simulink model "AMR_main_24a"  (R2024a)
settings: configuration reference "SharedConfig" (kept outside this file)
values from neighbouring files (symbols this model uses):
  tstep = 0.001    [configuration_dictionary.sldd]
undefined symbols (not defined in the file or in its folder): Down, Pull, RTK_health_condition
libraries: speedgoatlib_IO60X_IO69X x11, tramontina_database_nvidialib x11, tramontina_database_curtislib x9, slrealtimeiplib x5, tramontina_database_curtis_mesalib x2, tramontina_database_moboticlib x2, speedgoatlib_IO691 x2, slrealtimeloglib x2, tramontina_database_sick_modbuslib x1, canmsglib x1, slrealtimeptplib x1
(part 1 of 2)
settings Model: DataDictionary=configuration_dictionary.sldd  SimulationMode=external  ExtModeEnableFloating=off  ExtModeTrigDuration=100000  Creator=matlab.cut  LastModifiedBy=matlab.cut
settings ConfigSetRef: SourceName=SharedConfig

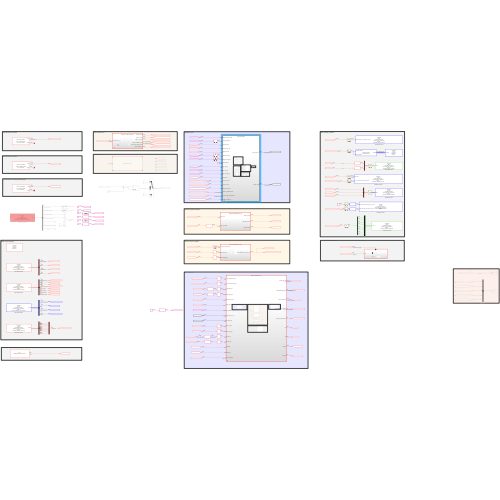
[thumbnail: Simulink's stored preview of the top-level diagram]
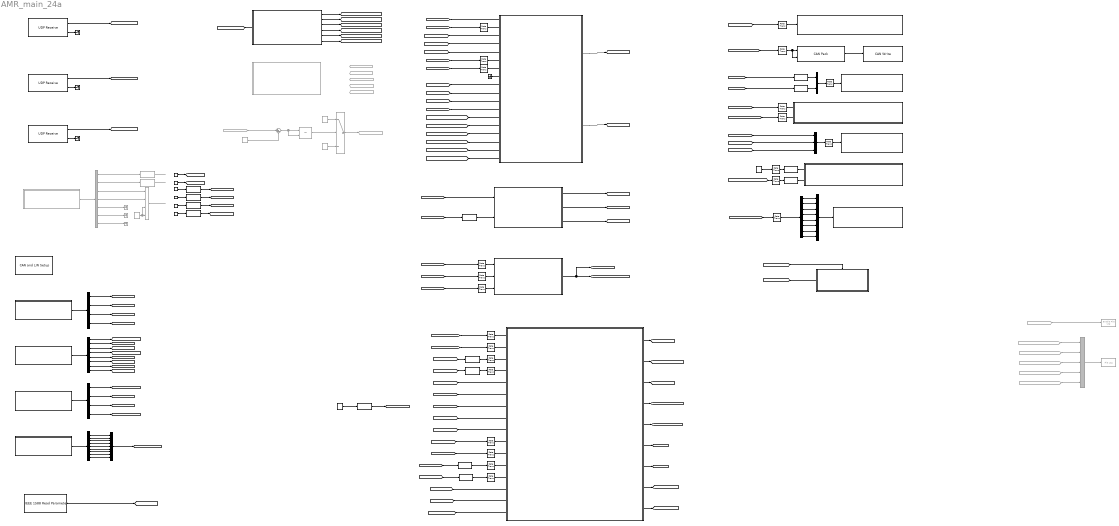
== system AMR_main_24a ==
  note: LidarLoc UPD Decoder
  note: Read UDP Data from Joystick
  note: Write UDP Data to LidarLoc Odometry
  note: Read System Time
  note: Motor Controll Untit
  note: guidance_unit
  note: operation_mode_selector
  note: vehicle_speed_readout
  note: CAN_output_interface
  note: CAN_input_interface
  note: Read UDP Data from Joystick
  note: gnss UPD Decoder
  note: Read UDP Data from ArduSimple Heading gnss
  Bus Creator : BusCreator  Inputs=8
  Bus Creator1 : BusCreator  Commented=on  Inputs=5
  Bus Creator2 : BusCreator  Inputs=2
  Bus Creator3 : BusCreator  Inputs=3
  Bus Selector1 : BusSelector  OutputSignals=ID1832_controller_status_RCUfront.controller_mode_front,ID1832_controller_status_RCUfront.MessageStatus.Status,ID1833_controller_status_RCUrear.controller_mode_rear,ID1833_controller_status_RCUrear.MessageStatus.Status
  Bus Selector6 : BusSelector  OutputSignals=ID1830_controller_status_left.controller_mode_left,ID1830_controller_status_left.MessageStatus.Status,ID1831_controller_status_right.MessageStatus.Status,ID1831_controller_status_right.controller_mode_right,ID422_curtis_feedback_message_left.motor_rpm_left,ID423_curtis_feedback_message_right.motor_rpm_right,ID934_curtis_encoder_left.rotor_position_left,ID935_curtis_encoder_right.rotor_position_rigth
  Bus Selector7 : BusSelector  Commented=on  OutputSignals=ID341_read_from_flexisoft.AuxEmEmergencia,ID341_read_from_flexisoft.AuxScannerInterrompido,ID341_read_from_flexisoft.EmergenciaFrontalDireita,ID341_read_from_flexisoft.EmergenciaFrontalEsquerda,ID341_read_from_flexisoft.EmergenciaTraseiraDireita,ID341_read_from_flexisoft.EmergenciaTraseiraEsquerda,ID341_read_from_flexisoft.MessageStatus.Status
  Bus Selector8 : BusSelector  OutputSignals=ID1459_feedback_word.MessageStatus.Status,ID1459_feedback_word.byte0,ID1459_feedback_word.byte1,ID1459_feedback_word.byte2,ID1459_feedback_word.byte3,ID1459_feedback_word.byte4,ID1459_feedback_word.byte5,ID1459_feedback_word.byte6,ID1459_feedback_word.byte7
  Bus Selector9 : BusSelector  OutputSignals=ID288_mobotic_feedback_pos.position_feedback,ID288_mobotic_feedback_pos.MessageStatus.Status,ID343_AMR_OperationMode.OperationMode,ID343_AMR_OperationMode.MessageStatus.Status
  CAN DB Parser Read 1 : Subsystem
      settings: OpenFcn=sg_can.OpenFcnRead;
      mask Help: eval('sg.utils.help.show(''io_main/refentry_ref_can_ofa_parsing_read'');')
      mask Display: disp('Speedgoat\nIO691\nCAN DB Parser Read\nModule ID: IO691 - Module ID 1\nChannel:  1\ntramontina_database_curtis_mesa.dbc ');
  CAN DB Parser Read 3 : Subsystem
      settings: OpenFcn=sg_can.OpenFcnRead;
      mask Help: eval('sg.utils.help.show(''io_main/refentry_ref_can_ofa_parsing_read'');')
      mask Display: disp('Speedgoat\nIO691\nCAN DB Parser Read\nModule ID: IO691 - Module ID 1\nChannel:  1\ntramontina_database_curtis.dbc ');
  CAN DB Parser Read 4 : Subsystem  Commented=on
      settings: OpenFcn=sg_can.OpenFcnRead;
      mask Help: eval('sg.utils.help.show(''io_main/refentry_ref_can_ofa_parsing_read'');')
      mask Display: disp('Speedgoat\nIO691\nCAN DB Parser Read\nModule ID: IO691 - Module ID 1\nChannel:  1\ntramontina_database_sick_modbus.dbc ');
  CAN DB Parser Read 7 : Subsystem
      settings: OpenFcn=sg_can.OpenFcnRead;
      mask Help: eval('sg.utils.help.show(''io_main/refentry_ref_can_ofa_parsing_read'');')
      mask Display: disp('Speedgoat\nIO691\nCAN DB Parser Read\nModule ID: IO691 - Module ID 1\nChannel:  1\ntramontina_database_mobotic.dbc ');
  CAN DB Parser Read 9 : Subsystem
      settings: OpenFcn=sg_can.OpenFcnRead;
      mask Help: eval('sg.utils.help.show(''io_main/refentry_ref_can_ofa_parsing_read'');')
      mask Display: disp('Speedgoat\nIO691\nCAN DB Parser Read\nModule ID: IO691 - Module ID 1\nChannel:  1\ntramontina_database_nvidia.dbc ');
  "CAN DB Parser Write " : Subsystem
      settings: OpenFcn=sg_can.OpenFcnWrite;
      mask Help: eval('sg.utils.help.show(''io_main/refentry_ref_can_ofa_parsing_write'');')
      mask Display: disp('Speedgoat\nIO691\nCAN DB Parser Write\nModule ID: IO691 - Module ID 1\nChannel:  1\ntramontina_database_nvidia.dbc ');
  CAN DB Parser Write 1 : Subsystem
      settings: OpenFcn=sg_can.OpenFcnWrite;
      mask Help: eval('sg.utils.help.show(''io_main/refentry_ref_can_ofa_parsing_write'');')
      mask Display: disp('Speedgoat\nIO691\nCAN DB Parser Write\nModule ID: IO691 - Module ID 1\nChannel:  1\ntramontina_database_nvidia.dbc ');
  CAN DB Parser Write 2 : Subsystem
      settings: OpenFcn=sg_can.OpenFcnWrite;
      mask Help: eval('sg.utils.help.show(''io_main/refentry_ref_can_ofa_parsing_write'');')
      mask Display: disp('Speedgoat\nIO691\nCAN DB Parser Write\nModule ID: IO691 - Module ID 1\nChannel:  1\ntramontina_database_curtis.dbc ');
  CAN DB Parser Write 3 : Subsystem
      settings: OpenFcn=sg_can.OpenFcnWrite;
      mask Help: eval('sg.utils.help.show(''io_main/refentry_ref_can_ofa_parsing_write'');')
      mask Display: disp('Speedgoat\nIO691\nCAN DB Parser Write\nModule ID: IO691 - Module ID 1\nChannel:  1\ntramontina_database_curtis.dbc ');
  CAN DB Parser Write 5 : Subsystem
      settings: OpenFcn=sg_can.OpenFcnWrite;
      mask Help: eval('sg.utils.help.show(''io_main/refentry_ref_can_ofa_parsing_write'');')
      mask Display: disp('Speedgoat\nIO691\nCAN DB Parser Write\nModule ID: IO691 - Module ID 1\nChannel:  1\ntramontina_database_nvidia.dbc ');
  CAN DB Parser Write 6 : Subsystem
      settings: OpenFcn=sg_can.OpenFcnWrite;
      mask Help: eval('sg.utils.help.show(''io_main/refentry_ref_can_ofa_parsing_write'');')
      mask Display: disp('Speedgoat\nIO691\nCAN DB Parser Write\nModule ID: IO691 - Module ID 1\nChannel:  1\ntramontina_database_mobotic.dbc ');
  CAN Pack2 : canmsglib/CAN Pack  MsgList=(none)  MsgName=CAN Msg  MsgIDType=Standard (11-bit identifier)  MsgIdentifier=0x120  MsgLength=8  Remote=off  ApplyMinMax=off  BusOutput=on  SignalInfo={ 'position_feedback', '0', '32', 'LE', 'signed', 'Standard', '0', '1', '0', '-inf', 'inf'; 'pulse_feedback', '32', '32', 'LE', 'signed', 'Standard', '0', '1', '0', '-Inf', 'Inf' }
      settings: DataFormat=manually specified signals
  CAN Write 2 : speedgoatlib_IO691/CAN Write   moduleType=IO691  id=1  channel=1  canType=CAN (HS)  messageType=CAN (HS)  useBusIn=on  numOfMsg=1  enableInput=off  enableStatusPort=off  ts=20e-3  initValues=[691 1 0.02 0 1 1 0 1 0 1]
      settings: SourceProductName=IO691
  "CAN and LIN Setup " : speedgoatlib_IO691/CAN and LIN Setup   moduleInitValues="[691    1    1   -1   -1]"  id=1  moduleType=IO691  pciSlot=-1  canChn1=CAN (HS)  canChn2=Disabled  canChn3=Disabled  canChn4=Disabled  linChn1=Disabled  linChn2=Disabled  canInitStructArray=[]  canTermStructArray=[]  gpioChnx=Disabled  canChn1InitValues="[2   2   8   1  16   3  19   2   2   5   2   0]"  arbBdrChn1=500 kBaud  clockDividerChn1=Enable  arbManBdrChn1=[8,1,16,3]  fdBdrChn1=5.0 MBaud  fdManBdrChn1=[2,2,5,2]  termResistor1=off  canChn2InitValues="[1   0   2   8  31   8  19   2   2   5   2   0]"  arbBdrChn2=1.0 MBaud  clockDividerChn2=Enable  arbManBdrChn2=[2,8,31,8]  fdBdrChn2=5.0 MBaud  fdManBdrChn2=[2,2,5,2]  termResistor2=off  canChn3InitValues="[1   0   2   8  31   8  19   2   2   5   2   0]"  arbBdrChn3=1.0 MBaud  clockDividerChn3=Enable  arbManBdrChn3=[2,8,31,8]  fdBdrChn3=5.0 MBaud  fdManBdrChn3=[2,2,5,2]  termResistor3=off  canChn4InitValues="[1   0   2   8  31   8  19   2   2   5   2   0]"  arbBdrChn4=1.0 MBaud  clockDividerChn4=Enable  arbManBdrChn4=[2,8,31,8]  fdBdrChn4=5.0 MBaud  fdManBdrChn4=[2,2,5,2]  termResistor4=off  linChn1InitValues="[0  9600]"  linBtrChn1=9600  linChn2InitValues="[0  9600]"  linBtrChn2=9600  doInitTermStruct="[0  5  0  0  0]"  parDoChannels=[1 2]  parDoVoltage=5  parDoInitValues=0  parDoReset=1  parNumOfDoS=0  parDiChannels=[3 4]  parDiVoltage=5  parDiPull=Pull-Down
      settings: LibrarySourceBlock=speedgoatlib_IO602_IO691/CAN and LIN Setup
  Cast{,1,4..9} (8 alike) : DataTypeConversion  OutDataTypeStr=boolean  SaturateOnIntegerOverflow=off  RndMeth=Floor
  Cast To Boolean : DataTypeConversion  Commented=on  OutDataTypeStr=boolean  SaturateOnIntegerOverflow=off  RndMeth=Floor
  Cast To Boolean1 : DataTypeConversion  Commented=on  OutDataTypeStr=boolean  SaturateOnIntegerOverflow=off  RndMeth=Floor
  Cast10 : DataTypeConversion  OutDataTypeStr=double  SaturateOnIntegerOverflow=off  RndMeth=Floor
  Cast11 : DataTypeConversion  OutDataTypeStr=double  SaturateOnIntegerOverflow=off  RndMeth=Floor
  Cast13 : DataTypeConversion  OutDataTypeStr=int64  SaturateOnIntegerOverflow=off  RndMeth=Floor
  Cast14 : DataTypeConversion  OutDataTypeStr=int64  SaturateOnIntegerOverflow=off  RndMeth=Floor
  Cast2 : DataTypeConversion  OutDataTypeStr=single  SaturateOnIntegerOverflow=off  RndMeth=Floor
  Cast3 : DataTypeConversion  OutDataTypeStr=single  SaturateOnIntegerOverflow=off  RndMeth=Floor
  Constant : Constant  OutDataTypeStr=boolean
  Constant1 : Constant
  Constant10 : Constant  Commented=on
  Constant2 : Constant
  Constant3 : Constant  Value=0
  Constant4 : Constant
  Constant5 : Constant  Value=0
  Constant8 : Constant  Commented=on
  Constant9 : Constant  Commented=on  Value=0
  Demux1 : Demux  Outputs=8
  Enable File Log : slrealtimeloglib/Enable File Log  Commented=on
  Enabled Subsystem : Subsystem  TreatAsAtomicUnit=on
  File Log : slrealtimeloglib/File Log  Commented=on  decimation=1  inputProcessing=Elements as channels (sample based)
  From46 : From  Commented=on  GotoTag=GPS_RTKstatus
  From48 : From  Commented=on  GotoTag=LidarLoc_result_x
  From52 : From  Commented=on  GotoTag=LidarLoc_result_y
  From54 : From  Commented=on  GotoTag=LidarLoc_result_yaw
  From55 : From  Commented=on  GotoTag=LidarLoc_localization_status
  From56 : From  Commented=on  GotoTag=LidarLoc_map_matching_status
  From57 : From  Commented=on  GotoTag=AMR_auto_mode
  Goto22 : Goto  Commented=on  GotoTag=GPS_rtk_trustness
  Goto25 : Goto  Commented=on  GotoTag=GPS_RTKstatus
  Goto3 : Goto  Commented=on  GotoTag=gnss_lat_deg
  Goto4 : Goto  Commented=on  GotoTag=gnss_lon_deg
  Goto5 : Goto  Commented=on  GotoTag=gnss_heading_deg
  Goto9 : Goto  Commented=on  GotoTag=GPS_GNSSfix
  Ground : Ground
  IEEE 1588 Read Parameter : slrealtimeptplib/IEEE 1588 Read Parameter  Priority=1  ID=1  param=1. System time (nanosecond)  sample_time=tstep
  Integrator1 : Integrator  Commented=on  ExternalReset=either  UpperSaturationLimit=1  LowerSaturationLimit=0  WrappedStateUpperValue=30  WrappedStateLowerValue=0
  Model : ModelReference  ModelNameDialog=deployAMR_stateflow.slx  SimulationMode=Normal  ModelReferenceVersion=3.78
  Model1 : ModelReference  ModelNameDialog=AMR_OperationModeSelector_24a.slx  SimulationMode=Normal  ModelReferenceVersion=2.14
  Model2 : ModelReference  ModelNameDialog=AMR_LidarLoc_UDP_decoder_24a.slx  SimulationMode=Normal  ModelReferenceVersion=5.26
  Model3 : ModelReference  ModelNameDialog=AMR_VehicleSpeedReadout_24a.slx  SimulationMode=Normal  ModelReferenceVersion=2.16
  Model4 : ModelReference  ModelNameDialog=AMR_MotorControlUnit_24a.slx  SimulationMode=Normal  ModelReferenceVersion=2.51
      settings: PortSchema="{\"entries\":[{\"content\":{\"sides\":[{\"content\":{\"connectorIds\":[\"In1\",\"In2\",\"In3\",\"In4\",\"In6\",\"In7\",\"In8\",\"In9\",\"In10\",\"In11\",\"In12\",\"In13\",\"In14\",\"In15\",\"In5\",\"In16\"]},\"type\":\"ConnectorPlacement.EquallySpacedRectSide\",\"uuid\":\"7c2b178d-2b94-42de-b877-cc3b9587523f\"},{\"content\":{\"connectorIds\":[\"Out1\",\"Out2\",\"Out3\",\"Out4\",\"Out5\",\"Out6\",\"Out7\",\"Out8\",\"Out9\"],\"side\":\"RIGHT\"},\"type\":\"ConnectorPlacement.EquallySpacedRectSide\",\"uuid\":\"578e4da8-0cd4-4538-9680-61a080b2bcd8\"},{\"content\":{\"side\":\"TOP\"},\"type\":\"ConnectorPlacement.EquallySpacedRectSide\",\"uuid\":\"8fde1a66-cc00-48a8-a863-0a641ec024c7\"}]},\"type\":\"ConnectorPlacement.EquallySpacedConnector\",\"uuid\":\"3439c5b0-61a5-4e62-aad1-c2c681181905\"}],\"packageUris\":[\"http://schema.mathworks.com/mf0/Connector/R2020b\"],\"version\":\"1.0\"}"
  Model5 : ModelReference  Commented=on  SimulationMode=Normal
  Mux : Mux  Inputs=9
  OR : Logic  Commented=on  Operator=OR  Inputs=4  AllPortsSameDT=off  OutDataTypeStr=boolean
  Rate Transition{,1..2,6,9..10,15,22..24,26,28..29,32,38,40..44} (20 alike) : RateTransition
  Rate Transition11 : RateTransition  OutPortSampleTimeOpt=Inherit
  Rate Transition12 : RateTransition  Deterministic=off
  Rate Transition21 : RateTransition  OutPortSampleTimeOpt=Inherit
  Sum1 : Sum  Commented=on  Inputs=|+-
  Switch2 : Switch  Commented=on  Criteria=u2 > Threshold  Threshold=RTK_health_condition  SaturateOnIntegerOverflow=off  InputSameDT=off
  Terminator : Terminator  Commented=on
  Terminator1 : Terminator  Commented=on
  Terminator2 : Terminator  Commented=on
  Terminator3 : Terminator
  Terminator4 : Terminator
  Terminator5 : Terminator
  UDP Receive : slrealtimeiplib/UDP Receive  useHostTargetConn=off  ipAddress=10.200.83.53  localPort=25000  rcvWidth=36  rcvFmAny=off  fmAddress='10.200.83.57'  sampleTime=tstep  enableMessage=off  maxPackets=1
  UDP Receive1 : slrealtimeiplib/UDP Receive  useHostTargetConn=off  ipAddress=10.200.83.53  localPort=5010  rcvWidth=56  rcvFmAny=on  fmAddress='10.200.83.57'  sampleTime=tstep  enableMessage=off  maxPackets=1
  UDP Receive2 : slrealtimeiplib/UDP Receive  useHostTargetConn=off  ipAddress=10.200.83.53  localPort=5015  rcvWidth=36  rcvFmAny=off  fmAddress='10.200.83.57'  sampleTime=tstep  enableMessage=off  maxPackets=1
  Zero : Constant  Commented=on  Value=0  OutDataTypeStr=Inherit: Inherit via back propagation
  Zero1 : Constant  Value=0  OutDataTypeStr=Inherit: Inherit via back propagation
  Zero2 : Constant  Value=0  OutDataTypeStr=Inherit: Inherit via back propagation
  wires:
  Rate Transition32/1 -> CAN DB Parser Write 5/1(ID289_mobotic_error_flag.steering_unit_error)
  Rate Transition28/1 -> Cast2/1
  [AMR_speed_to_CAN_m_per_sec] -> Rate Transition29/1
  Zero2/1 -> Rate Transition28/1
  CAN Pack2/1 -> CAN Write 2/1
  Bus Creator2/1 -> Rate Transition15/1
  [rws] -> Cast11/1  "rws"
  Cast10/1 -> Bus Creator2/1
  Rate Transition6/1 -> CAN DB Parser Write 3/2(ID0_curtis_input_operational.pre_operational)
  Bus Creator3/1 -> Rate Transition12/1
  [steering_unit_error] -> Rate Transition32/1
  Rate Transition10/1 -> CAN Pack2/2, CAN Pack2/1
  Rate Transition29/1 -> Cast3/1
  [curtis_controller_into_operation] -> Rate Transition6/1
  [lws] -> Cast10/1  "lws"
  Cast11/1 -> Bus Creator2/2
  [steering_unit_theta_position] -> Rate Transition10/1
  [controller_enable_flag] -> Rate Transition24/1
  Rate Transition15/1 -> CAN DB Parser Write 2/1(CAN Tx)
  Rate Transition24/1 -> CAN DB Parser Write 3/1(Enable Input)
  [interlock] -> Rate Transition44/1
  [emergency] -> Rate Transition43/1
  [scanner_blocked] -> Rate Transition42/1
  Rate Transition44/1 -> Model/2
  [gate_closed_ahead] -> Model/1
  Model/1 -> [target_speed_m_per_s]  "target_speed_m_s"
  Model/2 -> [sw_target_angle]  "sw_target_angle"
  Cast4/1 -> Model1/2
  Model1/1 -> [AMR_idle_mode]
  Model1/2 -> [AMR_manual_mode]
  Model1/3 -> [AMR_auto_mode]
  [curtis_controller_mode_left] -> Rate Transition21/1
  Rate Transition22/1 -> Model4/3
  Rate Transition21/1 -> Model4/1
  Rate Transition23/1 -> Model4/4
  Rate Transition11/1 -> Model4/2
  [curtis_status_right] -> Cast1/1
  [curtis_status_left] -> Cast5/1
  [curtis_controller_mode_right] -> Rate Transition11/1
  [motor_rpm_right] -> Rate Transition41/1
  [steering_unit_pos] -> Rate Transition38/1
  [motor_rpm_left] -> Rate Transition40/1
  Model3/1 -> [AMR_speed_to_CAN_m_per_sec], [AMR_speed]
  Rate Transition38/1 -> Model3/1
  Rate Transition41/1 -> Model3/3
  Rate Transition40/1 -> Model3/2
  [motor_rpm_left] -> Rate Transition26/1
  [motor_rpm_right] -> Rate Transition9/1
  Cast2/1 -> CAN DB Parser Write 1/1(ID290_AMR_vehicle_speed.speed_m_per_min)
  Cast3/1 -> CAN DB Parser Write 1/2(ID290_AMR_vehicle_speed.speed_m_per_s)
  [AMR_idle_mode] -> Bus Creator3/1
  [AMR_auto_mode] -> Bus Creator3/3
  [AMR_manual_mode] -> Bus Creator3/2
  Cast5/1 -> Rate Transition22/1
  Cast1/1 -> Rate Transition23/1
  Rate Transition12/1 -> "CAN DB Parser Write "/1(CAN Tx)
  [oper_mode] -> Model1/1
  [oper_mode_status] -> Cast4/1
  Model4/1 -> [steering_unit_error]  "steering_unit_error"
  Model4/7 -> [rws]
  Bus Selector7/4 -> OR/2  "<EmergenciaFrontalEsquerda>"
  Zero/1 -> OR/3, OR/4
  Bus Selector9/4 -> [oper_mode_status]  "<Status>"
  Bus Selector9/3 -> [oper_mode]  "<OperationMode>"
  Cast To Boolean/1 -> ?
  CAN DB Parser Read 9/1(CAN Rx) -> Bus Selector9/1
  Bus Selector9/1 -> [steering_unit_pos]  "<position_feedback>"
  Bus Selector7/7 -> Terminator/1  "<Status>"
  Cast To Boolean1/1 -> ?
  Bus Selector7/1 -> Cast To Boolean/1  "<AuxEmEmergencia>"
  CAN DB Parser Read 4/1(CAN Rx) -> Bus Selector7/1
  CAN DB Parser Read 7/1(CAN Rx) -> Bus Selector8/1
  OR/1 -> ?  "emergency"
  Bus Selector7/2 -> Cast To Boolean1/1  "<AuxScannerInterrompido>"
  Bus Selector7/6 -> Terminator1/1  "<EmergenciaTraseiraEsquerda>"
  Bus Selector7/3 -> OR/1  "<EmergenciaFrontalDireita>"
  Bus Selector7/5 -> Terminator2/1  "<EmergenciaTraseiraDireita>"
  Bus Selector9/2 -> [steering_unit_status]  "<Status>"
  From46/1 -> Sum1/1
  Constant10/1 -> Sum1/2
  Constant9/1 -> Switch2/3
  Switch2/1 -> Goto22/1  "rtk_trustness"
  Integrator1/1 -> Switch2/2  "rtk_integrator"
  Constant8/1 -> Switch2/1
  Sum1/1 -> Integrator1/2, Integrator1/1  "rtk_diff"
  Rate Transition9/1 -> Model4/12
  [mobotic_Rx] -> Model4/5
  [AMR_manual_mode] -> Model4/6
  [AMR_auto_mode] -> Model4/7
  Demux1/8 -> Bus Creator/8
  Demux1/6 -> Bus Creator/6
  Demux1/4 -> Bus Creator/4
  Demux1/3 -> Bus Creator/3
  Demux1/5 -> Bus Creator/5
  Bus Creator/1 -> CAN DB Parser Write 6/1(CAN Tx)
  Demux1/7 -> Bus Creator/7
  [CANOpenMessage_Output] -> Rate Transition/1
  Rate Transition/1 -> Demux1/1
  Demux1/2 -> Bus Creator/2
  Demux1/1 -> Bus Creator/1
  Mux/1 -> [mobotic_Rx]  "mobotic_Rx"
  Bus Selector8/1 -> Mux/1  "<Status>"
  Bus Selector8/2 -> Mux/2  "<byte0>"
  Bus Selector8/3 -> Mux/3  "<byte1>"
  Bus Selector8/4 -> Mux/4  "<byte2>"
  Bus Selector8/5 -> Mux/5  "<byte3>"
  Bus Selector8/6 -> Mux/6  "<byte4>"
  Bus Selector8/7 -> Mux/7  "<byte5>"
  Bus Selector8/8 -> Mux/8  "<byte6>"
  Bus Selector8/9 -> Mux/9  "<byte7>"
  UDP Receive/2 -> Terminator4/1
  Model4/6 -> [lws]
  Model4/5 -> [steering_unit_theta_position]
  Model4/2 -> [CANOpenMessage_Output]  "CANOpenMessage_Output"
  Model4/3 -> [controller_enable_flag]  "controller_enable_flag"
  Model4/4 -> [curtis_controller_into_operation]  "curtis_controller_into_operation"
  Bus Selector1/3 -> [curtis_status_rear]  "<controller_mode_rear>"
  Bus Selector1/1 -> [curtis_controller_mode_front]  "<controller_mode_front>"
  Bus Selector1/4 -> [curtis_controller_mode_rear]  "<Status>"
  Bus Selector1/2 -> [curtis_status_front]  "<Status>"
  CAN DB Parser Read 1/1(CAN Rx) -> Bus Selector1/1
  Model4/8 -> [send_flag_odometry]
  Model4/9 -> [udp_string_odometry]
  [send_flag_odometry] -> Enabled Subsystem/Trigger  "sick_odometry_send_flag"
  [udp_string_odometry] -> Enabled Subsystem/1(data)  "udp_string"
  IEEE 1588 Read Parameter/1 -> [timestamp]  "output"
  [timestamp] -> Model4/15
  Bus Selector6/6 -> [motor_rpm_right]  "<motor_rpm_right>"
  Bus Selector6/5 -> [motor_rpm_left]  "<motor_rpm_left>"
  CAN DB Parser Read 3/1(CAN Rx) -> Bus Selector6/1
  Bus Selector6/8 -> [motor_encoder_right]  "<rotor_position_rigth>"
  Bus Selector6/2 -> [curtis_status_left]  "<Status>"
  Bus Selector6/4 -> [curtis_controller_mode_right]  "<controller_mode_right>"
  Bus Selector6/3 -> [curtis_status_right]  "<Status>"
  Bus Selector6/7 -> [motor_encoder_left]  "<rotor_position_left>"
  Bus Selector6/1 -> [curtis_controller_mode_left]  "<controller_mode_left>"
  Cast14/1 -> Rate Transition2/1
  Cast13/1 -> Rate Transition1/1  "encoder_left_int"
  [motor_encoder_right] -> Cast14/1
  [motor_encoder_left] -> Cast13/1  "encoder_left_double"
  Rate Transition1/1 -> Model4/13
  Rate Transition2/1 -> Model4/14
  UDP Receive/1 -> [udp_from_joystick]  "joy_axes"
  [udp_from_joystick] -> Model4/16
  [GPS_GNSSfix] -> Model4/8
  [target_speed_m_per_s] -> Model4/9
  [sw_target_angle] -> Model4/10
  Rate Transition26/1 -> Model4/11
  UDP Receive1/1 -> [udp_from_lidarLoc]  "udp_from_lidarLoc"
  UDP Receive1/2 -> Terminator3/1
  [udp_from_lidarLoc] -> Model2/1
  Model2/5 -> [LidarLoc_map_matching_status]
  Model2/4 -> [LidarLoc_localization_status]
  Model2/3 -> [LidarLoc_result_yaw]
  Model2/2 -> [LidarLoc_result_y]
  ? -> ?
  UDP Receive2/1 -> [udp_from_gnss]  "joy_axes"
  Constant/1 -> Cast/1
  Bus Creator1/1 -> File Log/1
  From48/1 -> Bus Creator1/1
  From52/1 -> Bus Creator1/2
  From54/1 -> Bus Creator1/3
  From55/1 -> Bus Creator1/4
  From56/1 -> Bus Creator1/5
  From57/1 -> Enable File Log/1  "auto_mode"
  Cast/1 -> [GPS_GNSSfix]
  Constant1/1 -> Cast6/1
  Constant3/1 -> Cast7/1
  Constant2/1 -> Cast8/1
  Model2/6 -> [LidarLoc_telegram_ok]
  Model2/1 -> [LidarLoc_result_x]
  [AMR_manual_mode] -> Model/4
  [AMR_auto_mode] -> Model/5
  [AMR_idle_mode] -> Model/3
  Rate Transition42/1 -> Model/6
  Rate Transition43/1 -> Model/7
  Ground/1 -> Model/8
  [gnss_lat_deg] -> Model/9
  [gnss_lon_deg] -> Model/10
  [gnss_heading_deg] -> Model/11
  [AMR_speed] -> Model/12
  [LidarLoc_result_x] -> Model/13
  [LidarLoc_result_y] -> Model/14
  [LidarLoc_result_yaw] -> Model/15
  [LidarLoc_localization_status] -> Model/16
  [LidarLoc_map_matching_status] -> Model/17
  [LidarLoc_telegram_ok] -> Model/18
  UDP Receive2/2 -> Terminator5/1
  Constant4/1 -> [one]
  Constant5/1 -> [nulo]
  Cast6/1 -> [interlock]
  Cast8/1 -> [emergency]
  Cast7/1 -> [scanner_blocked]
  Zero1/1 -> Cast9/1
  Cast9/1 -> [gate_closed_ahead]

== system AMR_main_24a/CAN DB Parser Read 1 ==
  ReadSubsystem : Subsystem
  UnpackSubsystem : Subsystem
  CAN Rx : Outport
  wires:
  ReadSubsystem/1(Raw_Rx) -> UnpackSubsystem/1(Unpack_In)
  ReadSubsystem/2(Status_Rx) -> UnpackSubsystem/2(Status Inport)
  UnpackSubsystem/1(Unpack_Out) -> CAN Rx/1

== system AMR_main_24a/CAN DB Parser Read 3 ==
  ReadSubsystem : Subsystem
  UnpackSubsystem : Subsystem
  CAN Rx : Outport
  wires:
  ReadSubsystem/1(Raw_Rx) -> UnpackSubsystem/1(Unpack_In)
  ReadSubsystem/2(Status_Rx) -> UnpackSubsystem/2(Status Inport)
  UnpackSubsystem/1(Unpack_Out) -> CAN Rx/1

== system AMR_main_24a/CAN DB Parser Read 4 ==
  ReadSubsystem : Subsystem
  UnpackSubsystem : Subsystem
  CAN Rx : Outport
  wires:
  ReadSubsystem/1(Raw_Rx) -> UnpackSubsystem/1(Unpack_In)
  ReadSubsystem/2(Status_Rx) -> UnpackSubsystem/2(Status Inport)
  UnpackSubsystem/1(Unpack_Out) -> CAN Rx/1

== system AMR_main_24a/CAN DB Parser Read 7 ==
  ReadSubsystem : Subsystem
  UnpackSubsystem : Subsystem
  CAN Rx : Outport
  wires:
  ReadSubsystem/1(Raw_Rx) -> UnpackSubsystem/1(Unpack_In)
  ReadSubsystem/2(Status_Rx) -> UnpackSubsystem/2(Status Inport)
  UnpackSubsystem/1(Unpack_Out) -> CAN Rx/1

== system AMR_main_24a/CAN DB Parser Read 9 ==
  ReadSubsystem : Subsystem
  UnpackSubsystem : Subsystem
  CAN Rx : Outport
  wires:
  ReadSubsystem/1(Raw_Rx) -> UnpackSubsystem/1(Unpack_In)
  ReadSubsystem/2(Status_Rx) -> UnpackSubsystem/2(Status Inport)
  UnpackSubsystem/1(Unpack_Out) -> CAN Rx/1

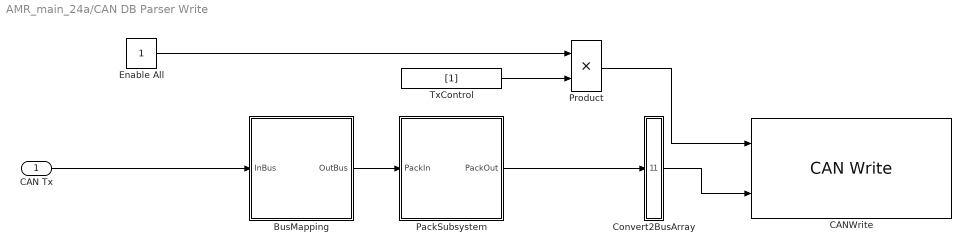
== system AMR_main_24a/CAN DB Parser Write  ==
  CAN Tx : Inport
  BusMapping : Subsystem
  CANWrite : speedgoatlib_IO60X_IO69X/CAN/CAN Write   moduleType=IO691  id=1  channel=1  canType=CAN (HS)  messageType=CAN (HS)  useBusIn=on  numOfMsg=1  enableInput=on  enableStatusPort=off  ts=500e-3  initValues=[691 1 0.5 0 1 1 0 1 1 1]
  Convert2BusArray : Subsystem
  Enable All : Constant  OutDataTypeStr=boolean
  PackSubsystem : Subsystem
  Product : Product  OutDataTypeStr=uint32
  TxControl : Constant  Value=[1]  OutDataTypeStr=uint32
  wires:
  PackSubsystem/1(PackOut) -> Convert2BusArray/1(InBus)
  Convert2BusArray/1(BusArrayOut) -> CANWrite/2
  Product/1 -> CANWrite/1
  TxControl/1 -> Product/2
  Enable All/1 -> Product/1
  CAN Tx/1 -> BusMapping/1(InBus)
  BusMapping/1(OutBus) -> PackSubsystem/1(PackIn)

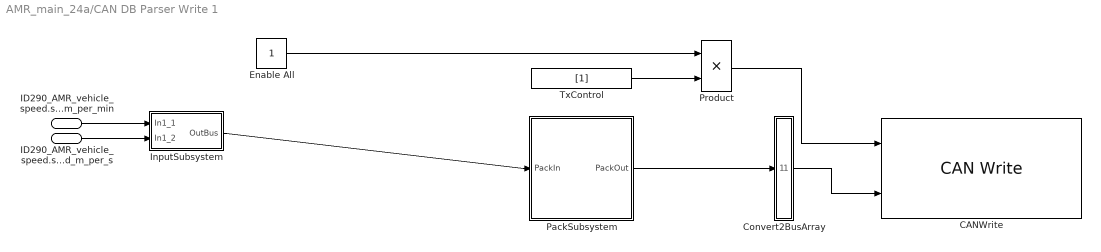
== system AMR_main_24a/CAN DB Parser Write 1 ==
  ID290_AMR_vehicle_speed.speed_m_per_min : Inport
  ID290_AMR_vehicle_speed.speed_m_per_s : Inport  Port=2
  CANWrite : speedgoatlib_IO60X_IO69X/CAN/CAN Write   moduleType=IO691  id=1  channel=1  canType=CAN (HS)  messageType=CAN (HS)  useBusIn=on  numOfMsg=1  enableInput=on  enableStatusPort=off  ts=50e-3  initValues=[691 1 0.05 0 1 1 0 1 1 1]
  Convert2BusArray : Subsystem
  Enable All : Constant  OutDataTypeStr=boolean
  InputSubsystem : Subsystem
  PackSubsystem : Subsystem
  Product : Product  OutDataTypeStr=uint32
  TxControl : Constant  Value=[1]  OutDataTypeStr=uint32
  wires:
  PackSubsystem/1(PackOut) -> Convert2BusArray/1(InBus)
  Convert2BusArray/1(BusArrayOut) -> CANWrite/2
  Product/1 -> CANWrite/1
  TxControl/1 -> Product/2
  Enable All/1 -> Product/1
  ID290_AMR_vehicle_speed.speed_m_per_min/1 -> InputSubsystem/1(In1_1)
  ID290_AMR_vehicle_speed.speed_m_per_s/1 -> InputSubsystem/2(In1_2)
  InputSubsystem/1(OutBus) -> PackSubsystem/1(PackIn)

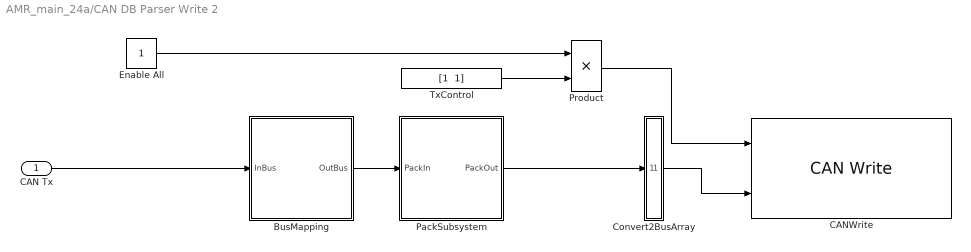
== system AMR_main_24a/CAN DB Parser Write 2 ==
  CAN Tx : Inport
  BusMapping : Subsystem
  CANWrite : speedgoatlib_IO60X_IO69X/CAN/CAN Write   moduleType=IO691  id=1  channel=1  canType=CAN (HS)  messageType=CAN (HS)  useBusIn=on  numOfMsg=2  enableInput=on  enableStatusPort=off  ts=10e-3  initValues=[691 1 0.01 0 1 1 0 2 1 1]
  Convert2BusArray : Subsystem
  Enable All : Constant  OutDataTypeStr=boolean
  PackSubsystem : Subsystem
  Product : Product  OutDataTypeStr=uint32
  TxControl : Constant  Value="[1  1]"  OutDataTypeStr=uint32
  wires:
  PackSubsystem/1(PackOut) -> Convert2BusArray/1(InBus)
  Convert2BusArray/1(BusArrayOut) -> CANWrite/2
  Product/1 -> CANWrite/1
  TxControl/1 -> Product/2
  Enable All/1 -> Product/1
  CAN Tx/1 -> BusMapping/1(InBus)
  BusMapping/1(OutBus) -> PackSubsystem/1(PackIn)

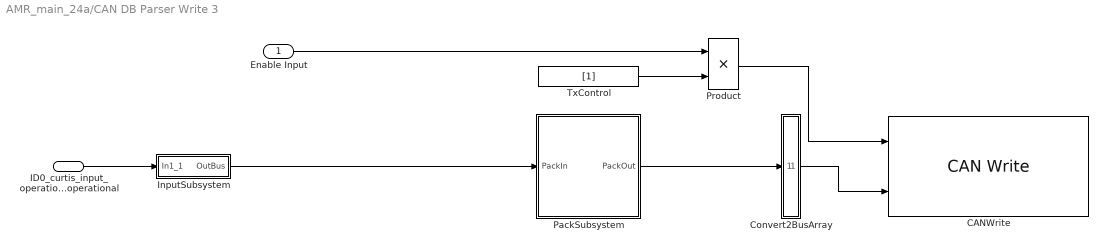
== system AMR_main_24a/CAN DB Parser Write 3 ==
  Enable Input : Inport  OutDataTypeStr=boolean
  ID0_curtis_input_operational.pre_operational : Inport  Port=2
  CANWrite : speedgoatlib_IO60X_IO69X/CAN/CAN Write   moduleType=IO691  id=1  channel=1  canType=CAN (HS)  messageType=CAN (HS)  useBusIn=on  numOfMsg=1  enableInput=on  enableStatusPort=off  ts=500e-3  initValues=[691 1 0.5 0 1 1 0 1 1 1]
  Convert2BusArray : Subsystem
  InputSubsystem : Subsystem
  PackSubsystem : Subsystem
  Product : Product  OutDataTypeStr=uint32
  TxControl : Constant  Value=[1]  OutDataTypeStr=uint32
  wires:
  PackSubsystem/1(PackOut) -> Convert2BusArray/1(InBus)
  Convert2BusArray/1(BusArrayOut) -> CANWrite/2
  Product/1 -> CANWrite/1
  TxControl/1 -> Product/2
  Enable Input/1 -> Product/1
  ID0_curtis_input_operational.pre_operational/1 -> InputSubsystem/1(In1_1)
  InputSubsystem/1(OutBus) -> PackSubsystem/1(PackIn)

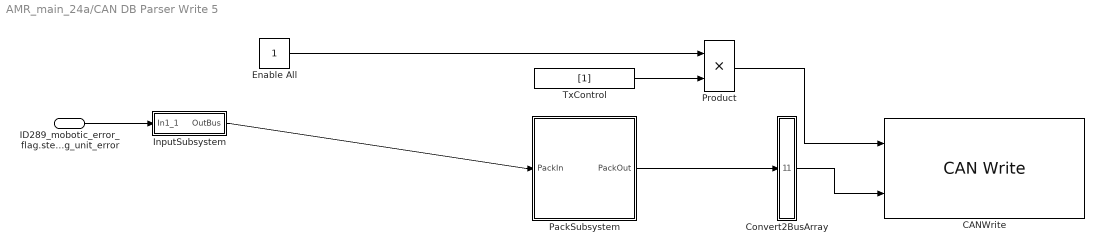
== system AMR_main_24a/CAN DB Parser Write 5 ==
  ID289_mobotic_error_flag.steering_unit_error : Inport
  CANWrite : speedgoatlib_IO60X_IO69X/CAN/CAN Write   moduleType=IO691  id=1  channel=1  canType=CAN (HS)  messageType=CAN (HS)  useBusIn=on  numOfMsg=1  enableInput=on  enableStatusPort=off  ts=500e-3  initValues=[691 1 0.5 0 1 1 0 1 1 1]
  Convert2BusArray : Subsystem
  Enable All : Constant  OutDataTypeStr=boolean
  InputSubsystem : Subsystem
  PackSubsystem : Subsystem
  Product : Product  OutDataTypeStr=uint32
  TxControl : Constant  Value=[1]  OutDataTypeStr=uint32
  wires:
  PackSubsystem/1(PackOut) -> Convert2BusArray/1(InBus)
  Convert2BusArray/1(BusArrayOut) -> CANWrite/2
  Product/1 -> CANWrite/1
  TxControl/1 -> Product/2
  Enable All/1 -> Product/1
  ID289_mobotic_error_flag.steering_unit_error/1 -> InputSubsystem/1(In1_1)
  InputSubsystem/1(OutBus) -> PackSubsystem/1(PackIn)

== system AMR_main_24a/CAN DB Parser Write 6 ==
  CAN Tx : Inport
  BusMapping : Subsystem
  CANWrite : speedgoatlib_IO60X_IO69X/CAN/CAN Write   moduleType=IO691  id=1  channel=1  canType=CAN (HS)  messageType=CAN (HS)  useBusIn=on  numOfMsg=1  enableInput=on  enableStatusPort=off  ts=10e-3  initValues=[691 1 0.01 0 1 1 0 1 1 1]
  Convert2BusArray : Subsystem
  Enable All : Constant  OutDataTypeStr=boolean
  PackSubsystem : Subsystem
  Product : Product  OutDataTypeStr=uint32
  TxControl : Constant  Value=[1]  OutDataTypeStr=uint32
  wires:
  PackSubsystem/1(PackOut) -> Convert2BusArray/1(InBus)
  Convert2BusArray/1(BusArrayOut) -> CANWrite/2
  Product/1 -> CANWrite/1
  TxControl/1 -> Product/2
  Enable All/1 -> Product/1
  CAN Tx/1 -> BusMapping/1(InBus)
  BusMapping/1(OutBus) -> PackSubsystem/1(PackIn)

== system AMR_main_24a/Enabled Subsystem ==
  data : Inport
  Trigger : TriggerPort  VariantControl=(inherit)  PortDimensions=1
  UDP Send : slrealtimeiplib/UDP Send  useHostTargetConn=off  toAddress='10.200.83.69'  toPort=5009  sampleTime=-1  enableMessage=off
  UDP Send1 : slrealtimeiplib/UDP Send  useHostTargetConn=off  toAddress='10.200.83.63'  toPort=5009  sampleTime=-1  enableMessage=off
  Width : Width
  Width1 : Width
  wires:
  Width/1 -> UDP Send/2
  data/1 -> Width1/1, UDP Send1/1, Width/1, UDP Send/1
  Width1/1 -> UDP Send1/2

== system AMR_main_24a/CAN DB Parser Read 1/ReadSubsystem ==
  CANRead_Std : speedgoatlib_IO60X_IO69X/CAN/CAN Read   moduleType=IO691  id=1  channel=1  canType=CAN (HS)  messageType=CAN (HS)  useBusOut=on  HasMulRead=Specify by IDs  MsgIDlist="[1832  1833]"  isEFF=off  LabelInHex=off  enableInput=off  initValues=[691 1 0.05 0 1 1 0 1 2 0 2 1832 1833]  ts=50*tstep
  Data Type ConversionStd : DataTypeConversion  OutDataTypeStr=uint8  SaturateOnIntegerOverflow=off  RndMeth=Floor
  StdSelector_ : Selector  IndexOptions=Index vector (dialog)  Indices=1  OutputSizes=1
  StdSelector_1 : Selector  IndexOptions=Index vector (dialog)  Indices=2  OutputSizes=1
  Std_ : Outport  PortName=Raw_Rx  Element=Std.ID1832
  Std_1 : Outport  PortName=Raw_Rx  Element=Std.ID1833
  StdStatus_ : Outport  Port=2  PortName=Status_Rx  Element=Std.ID1832
  StdStatus_1 : Outport  Port=2  PortName=Status_Rx  Element=Std.ID1833
  wires:
  CANRead_Std/1 -> Data Type ConversionStd/1
  CANRead_Std/2 -> Std_/1
  CANRead_Std/3 -> Std_1/1
  Data Type ConversionStd/1 -> StdSelector_/1, StdSelector_1/1
  StdSelector_/1 -> StdStatus_/1
  StdSelector_1/1 -> StdStatus_1/1

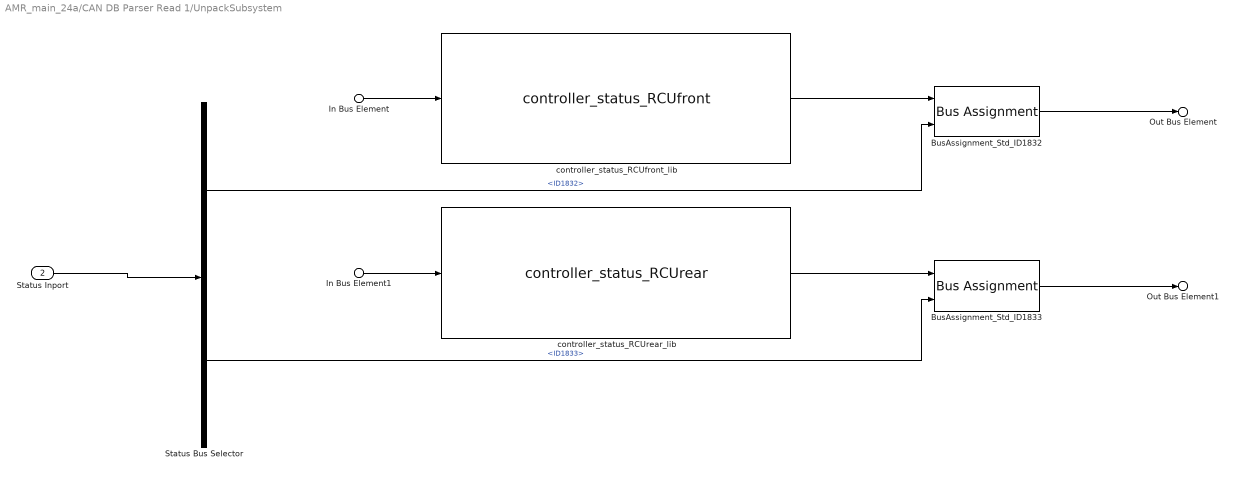
== system AMR_main_24a/CAN DB Parser Read 1/UnpackSubsystem ==
  In Bus Element : Inport  PortName=Unpack_In  Element=Std.ID1832
  In Bus Element1 : Inport  PortName=Unpack_In  Element=Std.ID1833
  Status Inport : Inport  Port=2
  BusAssignment_Std_ID1832 : BusAssignment  AssignedSignals=MessageStatus.Status
  BusAssignment_Std_ID1833 : BusAssignment  AssignedSignals=MessageStatus.Status
  Status Bus Selector : BusSelector  OutputSignals=Std.ID1832,Std.ID1833
  controller_status_RCUfront_lib : tramontina_database_curtis_mesalib/CAN unpack/controller_status_RCUfront  SystemSampleTime=-1  VariantActivationTime=update diagram  AllowFlexibleInterface=on  Latency=0  AutoFrameSizeCalculation=off
  controller_status_RCUrear_lib : tramontina_database_curtis_mesalib/CAN unpack/controller_status_RCUrear  SystemSampleTime=-1  VariantActivationTime=update diagram  AllowFlexibleInterface=on  Latency=0  AutoFrameSizeCalculation=off
  Out Bus Element : Outport  PortName=Unpack_Out  Element=ID1832_controller_status_RCUfront
  Out Bus Element1 : Outport  PortName=Unpack_Out  Element=ID1833_controller_status_RCUrear
  wires:
  In Bus Element/1 -> controller_status_RCUfront_lib/1
  controller_status_RCUfront_lib/1 -> BusAssignment_Std_ID1832/1
  BusAssignment_Std_ID1832/1 -> Out Bus Element/1
  In Bus Element1/1 -> controller_status_RCUrear_lib/1
  controller_status_RCUrear_lib/1 -> BusAssignment_Std_ID1833/1
  BusAssignment_Std_ID1833/1 -> Out Bus Element1/1
  Status Inport/1 -> Status Bus Selector/1
  Status Bus Selector/1 -> BusAssignment_Std_ID1832/2  "<ID1832>"
  Status Bus Selector/2 -> BusAssignment_Std_ID1833/2  "<ID1833>"

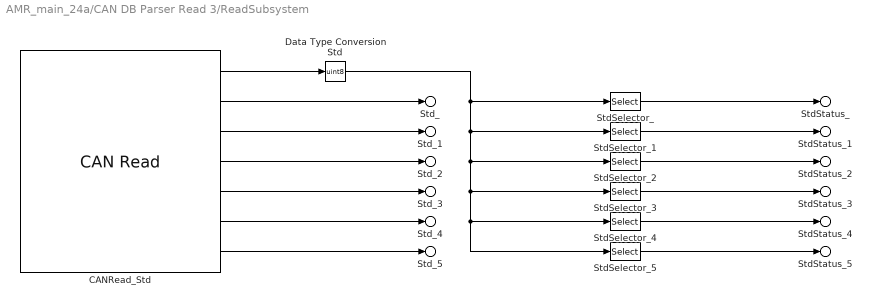
== system AMR_main_24a/CAN DB Parser Read 3/ReadSubsystem ==
  CANRead_Std : speedgoatlib_IO60X_IO69X/CAN/CAN Read   moduleType=IO691  id=1  channel=1  canType=CAN (HS)  messageType=CAN (HS)  useBusOut=on  HasMulRead=Specify by IDs  MsgIDlist="[422   423   934   935  1830  1831]"  isEFF=off  LabelInHex=off  enableInput=off  initValues=[691 1 0.001 0 1 1 0 1 2 0 6 422 423 934 935 1830 1831]  ts=tstep
  Data Type ConversionStd : DataTypeConversion  OutDataTypeStr=uint8  SaturateOnIntegerOverflow=off  RndMeth=Floor
  StdSelector_ : Selector  IndexOptions=Index vector (dialog)  Indices=1  OutputSizes=1
  StdSelector_1 : Selector  IndexOptions=Index vector (dialog)  Indices=2  OutputSizes=1
  StdSelector_2 : Selector  IndexOptions=Index vector (dialog)  Indices=3  OutputSizes=1
  StdSelector_3 : Selector  IndexOptions=Index vector (dialog)  Indices=4  OutputSizes=1
  StdSelector_4 : Selector  IndexOptions=Index vector (dialog)  Indices=5  OutputSizes=1
  StdSelector_5 : Selector  IndexOptions=Index vector (dialog)  Indices=6  OutputSizes=1
  Std_ : Outport  PortName=Raw_Rx  Element=Std.ID422
  Std_1 : Outport  PortName=Raw_Rx  Element=Std.ID423
  Std_2 : Outport  PortName=Raw_Rx  Element=Std.ID934
  Std_3 : Outport  PortName=Raw_Rx  Element=Std.ID935
  Std_4 : Outport  PortName=Raw_Rx  Element=Std.ID1830
  Std_5 : Outport  PortName=Raw_Rx  Element=Std.ID1831
  StdStatus_ : Outport  Port=2  PortName=Status_Rx  Element=Std.ID422
  StdStatus_1 : Outport  Port=2  PortName=Status_Rx  Element=Std.ID423
  StdStatus_2 : Outport  Port=2  PortName=Status_Rx  Element=Std.ID934
  StdStatus_3 : Outport  Port=2  PortName=Status_Rx  Element=Std.ID935
  StdStatus_4 : Outport  Port=2  PortName=Status_Rx  Element=Std.ID1830
  StdStatus_5 : Outport  Port=2  PortName=Status_Rx  Element=Std.ID1831
  wires:
  CANRead_Std/1 -> Data Type ConversionStd/1
  CANRead_Std/2 -> Std_/1
  CANRead_Std/3 -> Std_1/1
  CANRead_Std/4 -> Std_2/1
  CANRead_Std/5 -> Std_3/1
  CANRead_Std/6 -> Std_4/1
  CANRead_Std/7 -> Std_5/1
  Data Type ConversionStd/1 -> StdSelector_4/1, StdSelector_5/1, StdSelector_3/1, StdSelector_2/1, StdSelector_1/1, StdSelector_/1
  StdSelector_/1 -> StdStatus_/1
  StdSelector_1/1 -> StdStatus_1/1
  StdSelector_2/1 -> StdStatus_2/1
  StdSelector_3/1 -> StdStatus_3/1
  StdSelector_4/1 -> StdStatus_4/1
  StdSelector_5/1 -> StdStatus_5/1

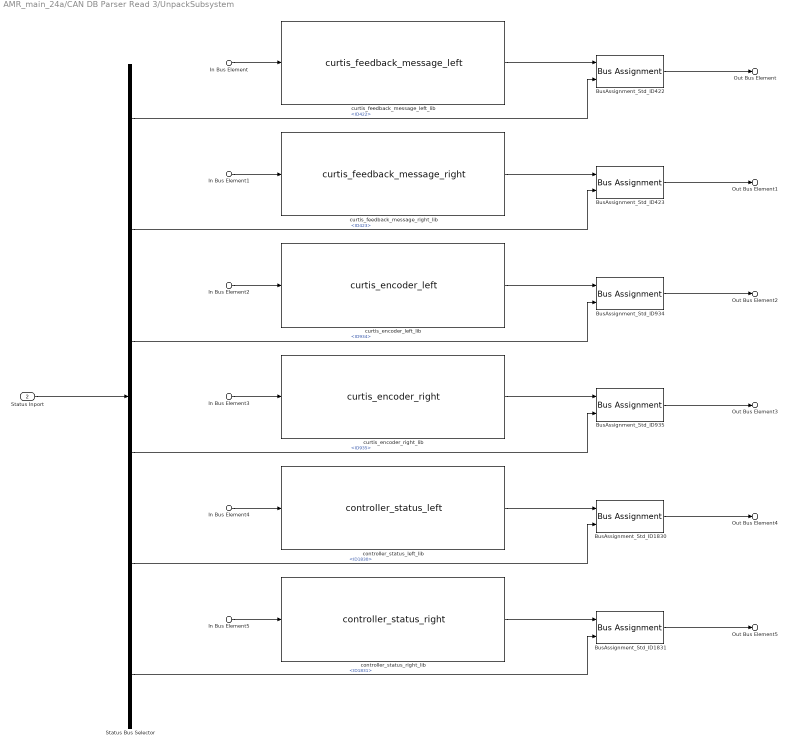
== system AMR_main_24a/CAN DB Parser Read 3/UnpackSubsystem ==
  In Bus Element : Inport  PortName=Unpack_In  Element=Std.ID422
  In Bus Element1 : Inport  PortName=Unpack_In  Element=Std.ID423
  In Bus Element2 : Inport  PortName=Unpack_In  Element=Std.ID934
  In Bus Element3 : Inport  PortName=Unpack_In  Element=Std.ID935
  In Bus Element4 : Inport  PortName=Unpack_In  Element=Std.ID1830
  In Bus Element5 : Inport  PortName=Unpack_In  Element=Std.ID1831
  Status Inport : Inport  Port=2
  BusAssignment_Std_ID{422..423,934..935,1830..1831} (6 alike) : BusAssignment  AssignedSignals=MessageStatus.Status
  Status Bus Selector : BusSelector  OutputSignals=Std.ID422,Std.ID423,Std.ID934,Std.ID935,Std.ID1830,Std.ID1831
  controller_status_left_lib : tramontina_database_curtislib/CAN unpack/controller_status_left  SystemSampleTime=-1  VariantActivationTime=update diagram  AllowFlexibleInterface=on  Latency=0  AutoFrameSizeCalculation=off
  controller_status_right_lib : tramontina_database_curtislib/CAN unpack/controller_status_right  SystemSampleTime=-1  VariantActivationTime=update diagram  AllowFlexibleInterface=on  Latency=0  AutoFrameSizeCalculation=off
  curtis_encoder_left_lib : tramontina_database_curtislib/CAN unpack/curtis_encoder_left  SystemSampleTime=-1  VariantActivationTime=update diagram  AllowFlexibleInterface=on  Latency=0  AutoFrameSizeCalculation=off
  curtis_encoder_right_lib : tramontina_database_curtislib/CAN unpack/curtis_encoder_right  SystemSampleTime=-1  VariantActivationTime=update diagram  AllowFlexibleInterface=on  Latency=0  AutoFrameSizeCalculation=off
  curtis_feedback_message_left_lib : tramontina_database_curtislib/CAN unpack/curtis_feedback_message_left  SystemSampleTime=-1  VariantActivationTime=update diagram  AllowFlexibleInterface=on  Latency=0  AutoFrameSizeCalculation=off
  curtis_feedback_message_right_lib : tramontina_database_curtislib/CAN unpack/curtis_feedback_message_right  SystemSampleTime=-1  VariantActivationTime=update diagram  AllowFlexibleInterface=on  Latency=0  AutoFrameSizeCalculation=off
  Out Bus Element : Outport  PortName=Unpack_Out  Element=ID422_curtis_feedback_message_left
  Out Bus Element1 : Outport  PortName=Unpack_Out  Element=ID423_curtis_feedback_message_right
  Out Bus Element2 : Outport  PortName=Unpack_Out  Element=ID934_curtis_encoder_left
  Out Bus Element3 : Outport  PortName=Unpack_Out  Element=ID935_curtis_encoder_right
  Out Bus Element4 : Outport  PortName=Unpack_Out  Element=ID1830_controller_status_left
  Out Bus Element5 : Outport  PortName=Unpack_Out  Element=ID1831_controller_status_right
  wires:
  In Bus Element/1 -> curtis_feedback_message_left_lib/1
  curtis_feedback_message_left_lib/1 -> BusAssignment_Std_ID422/1
  BusAssignment_Std_ID422/1 -> Out Bus Element/1
  In Bus Element1/1 -> curtis_feedback_message_right_lib/1
  curtis_feedback_message_right_lib/1 -> BusAssignment_Std_ID423/1
  BusAssignment_Std_ID423/1 -> Out Bus Element1/1
  In Bus Element2/1 -> curtis_encoder_left_lib/1
  curtis_encoder_left_lib/1 -> BusAssignment_Std_ID934/1
  BusAssignment_Std_ID934/1 -> Out Bus Element2/1
  In Bus Element3/1 -> curtis_encoder_right_lib/1
  curtis_encoder_right_lib/1 -> BusAssignment_Std_ID935/1
  BusAssignment_Std_ID935/1 -> Out Bus Element3/1
  In Bus Element4/1 -> controller_status_left_lib/1
  controller_status_left_lib/1 -> BusAssignment_Std_ID1830/1
  BusAssignment_Std_ID1830/1 -> Out Bus Element4/1
  In Bus Element5/1 -> controller_status_right_lib/1
  controller_status_right_lib/1 -> BusAssignment_Std_ID1831/1
  BusAssignment_Std_ID1831/1 -> Out Bus Element5/1
  Status Inport/1 -> Status Bus Selector/1
  Status Bus Selector/1 -> BusAssignment_Std_ID422/2  "<ID422>"
  Status Bus Selector/2 -> BusAssignment_Std_ID423/2  "<ID423>"
  Status Bus Selector/3 -> BusAssignment_Std_ID934/2  "<ID934>"
  Status Bus Selector/4 -> BusAssignment_Std_ID935/2  "<ID935>"
  Status Bus Selector/5 -> BusAssignment_Std_ID1830/2  "<ID1830>"
  Status Bus Selector/6 -> BusAssignment_Std_ID1831/2  "<ID1831>"

== system AMR_main_24a/CAN DB Parser Read 4/ReadSubsystem ==
  CANRead_Std : speedgoatlib_IO60X_IO69X/CAN/CAN Read   moduleType=IO691  id=1  channel=1  canType=CAN (HS)  messageType=CAN (HS)  useBusOut=on  HasMulRead=Specify by IDs  MsgIDlist=[341]  isEFF=off  LabelInHex=off  enableInput=off  initValues=[691 1 0.05 0 1 1 0 1 2 0 1 341]  ts=50*tstep
  Data Type ConversionStd : DataTypeConversion  OutDataTypeStr=uint8  SaturateOnIntegerOverflow=off  RndMeth=Floor
  StdSelector_ : Selector  IndexOptions=Index vector (dialog)  Indices=1  OutputSizes=1
  Std_ : Outport  PortName=Raw_Rx  Element=Std.ID341
  StdStatus_ : Outport  Port=2  PortName=Status_Rx  Element=Std.ID341
  wires:
  CANRead_Std/1 -> Data Type ConversionStd/1
  CANRead_Std/2 -> Std_/1
  Data Type ConversionStd/1 -> StdSelector_/1
  StdSelector_/1 -> StdStatus_/1

== system AMR_main_24a/CAN DB Parser Read 4/UnpackSubsystem ==
  In Bus Element : Inport  PortName=Unpack_In  Element=Std.ID341
  Status Inport : Inport  Port=2
  BusAssignment_Std_ID341 : BusAssignment  AssignedSignals=MessageStatus.Status
  Status Bus Selector : BusSelector  OutputSignals=Std.ID341
  read_from_flexisoft_lib : tramontina_database_sick_modbuslib/CAN unpack/read_from_flexisoft  SystemSampleTime=-1  VariantActivationTime=update diagram  AllowFlexibleInterface=on  Latency=0  AutoFrameSizeCalculation=off
  Out Bus Element : Outport  PortName=Unpack_Out  Element=ID341_read_from_flexisoft
  wires:
  In Bus Element/1 -> read_from_flexisoft_lib/1
  read_from_flexisoft_lib/1 -> BusAssignment_Std_ID341/1
  BusAssignment_Std_ID341/1 -> Out Bus Element/1
  Status Inport/1 -> Status Bus Selector/1
  Status Bus Selector/1 -> BusAssignment_Std_ID341/2  "<ID341>"

== system AMR_main_24a/CAN DB Parser Read 7/ReadSubsystem ==
  CANRead_Std : speedgoatlib_IO60X_IO69X/CAN/CAN Read   moduleType=IO691  id=1  channel=1  canType=CAN (HS)  messageType=CAN (HS)  useBusOut=on  HasMulRead=Specify by IDs  MsgIDlist=[1459]  isEFF=off  LabelInHex=off  enableInput=off  initValues=[691 1 0.001 0 1 1 0 1 2 0 1 1459]  ts=tstep
  Data Type ConversionStd : DataTypeConversion  OutDataTypeStr=uint8  SaturateOnIntegerOverflow=off  RndMeth=Floor
  StdSelector_ : Selector  IndexOptions=Index vector (dialog)  Indices=1  OutputSizes=1
  Std_ : Outport  PortName=Raw_Rx  Element=Std.ID1459
  StdStatus_ : Outport  Port=2  PortName=Status_Rx  Element=Std.ID1459
  wires:
  CANRead_Std/1 -> Data Type ConversionStd/1
  CANRead_Std/2 -> Std_/1
  Data Type ConversionStd/1 -> StdSelector_/1
  StdSelector_/1 -> StdStatus_/1

== system AMR_main_24a/CAN DB Parser Read 7/UnpackSubsystem ==
  In Bus Element : Inport  PortName=Unpack_In  Element=Std.ID1459
  Status Inport : Inport  Port=2
  BusAssignment_Std_ID1459 : BusAssignment  AssignedSignals=MessageStatus.Status
  Status Bus Selector : BusSelector  OutputSignals=Std.ID1459
  feedback_word_lib : tramontina_database_moboticlib/CAN unpack/feedback_word  SystemSampleTime=-1  VariantActivationTime=update diagram  AllowFlexibleInterface=on  Latency=0  AutoFrameSizeCalculation=off
  Out Bus Element : Outport  PortName=Unpack_Out  Element=ID1459_feedback_word
  wires:
  In Bus Element/1 -> feedback_word_lib/1
  feedback_word_lib/1 -> BusAssignment_Std_ID1459/1
  BusAssignment_Std_ID1459/1 -> Out Bus Element/1
  Status Inport/1 -> Status Bus Selector/1
  Status Bus Selector/1 -> BusAssignment_Std_ID1459/2  "<ID1459>"

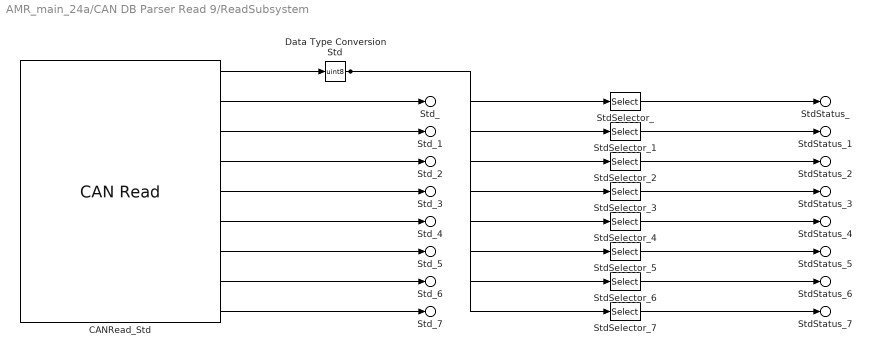
== system AMR_main_24a/CAN DB Parser Read 9/ReadSubsystem ==
  CANRead_Std : speedgoatlib_IO60X_IO69X/CAN/CAN Read   moduleType=IO691  id=1  channel=1  canType=CAN (HS)  messageType=CAN (HS)  useBusOut=on  HasMulRead=Specify by IDs  MsgIDlist="[288  343  368  369  370  371  372  373]"  isEFF=off  LabelInHex=off  enableInput=off  initValues=[691 1 0.001 0 1 1 0 1 2 0 8 288 343 368 369 370 371 372 373]  ts=tstep
  Data Type ConversionStd : DataTypeConversion  OutDataTypeStr=uint8  SaturateOnIntegerOverflow=off  RndMeth=Floor
  StdSelector_ : Selector  IndexOptions=Index vector (dialog)  Indices=1  OutputSizes=1
  StdSelector_1 : Selector  IndexOptions=Index vector (dialog)  Indices=2  OutputSizes=1
  StdSelector_2 : Selector  IndexOptions=Index vector (dialog)  Indices=3  OutputSizes=1
  StdSelector_3 : Selector  IndexOptions=Index vector (dialog)  Indices=4  OutputSizes=1
  StdSelector_4 : Selector  IndexOptions=Index vector (dialog)  Indices=5  OutputSizes=1
  StdSelector_5 : Selector  IndexOptions=Index vector (dialog)  Indices=6  OutputSizes=1
  StdSelector_6 : Selector  IndexOptions=Index vector (dialog)  Indices=7  OutputSizes=1
  StdSelector_7 : Selector  IndexOptions=Index vector (dialog)  Indices=8  OutputSizes=1
  Std_ : Outport  PortName=Raw_Rx  Element=Std.ID288
  Std_1 : Outport  PortName=Raw_Rx  Element=Std.ID343
  Std_2 : Outport  PortName=Raw_Rx  Element=Std.ID368
  Std_3 : Outport  PortName=Raw_Rx  Element=Std.ID369
  Std_4 : Outport  PortName=Raw_Rx  Element=Std.ID370
  Std_5 : Outport  PortName=Raw_Rx  Element=Std.ID371
  Std_6 : Outport  PortName=Raw_Rx  Element=Std.ID372
  Std_7 : Outport  PortName=Raw_Rx  Element=Std.ID373
  StdStatus_ : Outport  Port=2  PortName=Status_Rx  Element=Std.ID288
  StdStatus_1 : Outport  Port=2  PortName=Status_Rx  Element=Std.ID343
  StdStatus_2 : Outport  Port=2  PortName=Status_Rx  Element=Std.ID368
  StdStatus_3 : Outport  Port=2  PortName=Status_Rx  Element=Std.ID369
  StdStatus_4 : Outport  Port=2  PortName=Status_Rx  Element=Std.ID370
  StdStatus_5 : Outport  Port=2  PortName=Status_Rx  Element=Std.ID371
  StdStatus_6 : Outport  Port=2  PortName=Status_Rx  Element=Std.ID372
  StdStatus_7 : Outport  Port=2  PortName=Status_Rx  Element=Std.ID373
  wires:
  CANRead_Std/1 -> Data Type ConversionStd/1
  CANRead_Std/2 -> Std_/1
  CANRead_Std/3 -> Std_1/1
  CANRead_Std/4 -> Std_2/1
  CANRead_Std/5 -> Std_3/1
  CANRead_Std/6 -> Std_4/1
  CANRead_Std/7 -> Std_5/1
  CANRead_Std/8 -> Std_6/1
  CANRead_Std/9 -> Std_7/1
  Data Type ConversionStd/1 -> StdSelector_/1, StdSelector_1/1, StdSelector_2/1, StdSelector_3/1, StdSelector_4/1, StdSelector_5/1, StdSelector_6/1, StdSelector_7/1
  StdSelector_/1 -> StdStatus_/1
  StdSelector_1/1 -> StdStatus_1/1
  StdSelector_2/1 -> StdStatus_2/1
  StdSelector_3/1 -> StdStatus_3/1
  StdSelector_4/1 -> StdStatus_4/1
  StdSelector_5/1 -> StdStatus_5/1
  StdSelector_6/1 -> StdStatus_6/1
  StdSelector_7/1 -> StdStatus_7/1
